simulink model "gaasikyte"  (R2020b)
settings: Solver=ode45  StartTime=0.0  StopTime=500.0  RelTol=1e-3  EnableMultiTasking=on
libraries: simulink x1
settings Model: Creator=andres  LastModifiedBy=risto
settings DataIOCC: LimitDataPoints=on  SaveFormat=Array  ReturnWorkspaceOutputs=off
settings OptimizationCC: LifeSpan=inf
settings DebuggingCC: UnderspecifiedInitializationDetection=Classic  MergeDetectMultiDrivingBlocksExec=none  StateNameClashWarn=warning  SFUnexpectedBacktrackingDiag=warning  SFNoUnconditionalDefaultTransitionDiag=warning  SFExecutionAtInitializationDiag=none  ArithmeticOperatorsInVariantConditions=warning
settings HardwareCC: ProdBitPerPointer=32  ProdBitPerSizeT=32  ProdBitPerPtrDiffT=32  ProdLargestAtomicFloat=None  ProdIntDivRoundTo=Undefined  ProdEndianess=Unspecified  ProdWordSize=32  ProdHWDeviceType=32-bit Generic
settings ModelReferenceCC: PropagateSignalLabelsOutOfModel=off
settings SFSimCC: SimUseLocalCustomCode=off  CustomCodeUndefinedFunction=UseInterfaceOnly
settings RTWCC: RTWUseLocalCustomCode=off
settings CodeAppCC: StateflowObjectComments=on
settings GRTTargetCC: TargetLangStandard=C89/C90 (ANSI)
settings ConfigComp: CovMetricSettings=dw  CovSaveCumulativeToWorkspaceVar=on  CovSaveSingleToWorkspaceVar=on  CovExternalEMLEnable=off

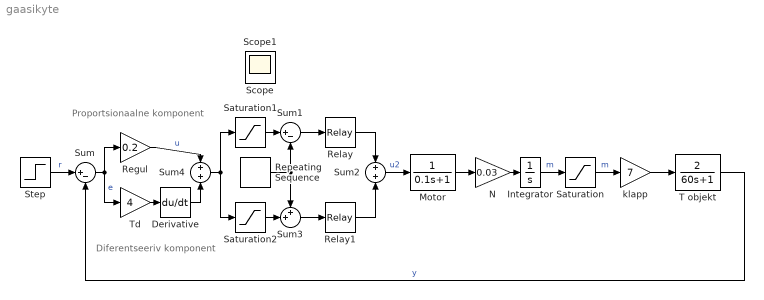
== system gaasikyte ==
  note: Diferentseeriv komponent
  note: Proportsionaalne komponent
  Derivative : Derivative
  Integrator : Integrator
  Motor : TransferFcn  Denominator=[0.1 1]
  N : Gain  Gain=0.03
  Regul : Gain  Gain=0.2
  Relay : Relay  OnSwitchValue=0  OffSwitchValue=-0.1  OnOutputValue=10
  Relay1 : Relay  OnSwitchValue=0  OffSwitchValue=-0.1  OnOutputValue=0  OffOutputValue=-10
  Repeating Sequence : simulink/Sources/Repeating Sequence  rep_seq_t=[0 10]  rep_seq_y=[0 10.1]
  Saturation : Saturate  UpperLimit=10  LowerLimit=0
  Saturation1 : Saturate  UpperLimit=10  LowerLimit=0
  Saturation2 : Saturate  UpperLimit=0  LowerLimit=-10
  Step : Step  Time=0  After=50  SampleTime=0
  Sum : Sum  Inputs=|+-
  Sum1 : Sum  Inputs=|+-
  Sum2 : Sum
  Sum3 : Sum  Inputs=++|
  Sum4 : Sum
  T objekt : TransferFcn  Numerator=[2]  Denominator=[60 1]
  Td : Gain  Gain=4
  klapp : Gain  Gain=7
  Scope : Scope
  Scope1 : Scope
  wires:
  Sum/1 -> Regul/1, Td/1  "e"
  Step/1 -> Sum/1  "r"
  T objekt/1 -> Sum/2  "y"
  klapp/1 -> T objekt/1
  Saturation/1 -> klapp/1  "m"
  Sum2/1 -> Motor/1  "u2"
  Repeating Sequence/1 -> Sum3/1, Sum1/2
  Saturation1/1 -> Sum1/1
  Sum1/1 -> Relay/1
  Relay/1 -> Sum2/1
  Motor/1 -> N/1
  Saturation2/1 -> Sum3/2
  Sum3/1 -> Relay1/1
  Relay1/1 -> Sum2/2
  N/1 -> Integrator/1
  Integrator/1 -> Saturation/1  "m"
  Td/1 -> Derivative/1
  Derivative/1 -> Sum4/2
  Regul/1 -> Sum4/1  "u"
  Sum4/1 -> Saturation2/1, Saturation1/1
